simulink model "motors"  (R2021b)
settings: Solver=VariableStepAuto  StartTime=0.0  StopTime=10.0  RelTol=1e-3
values from neighbouring files (symbols this model uses):
  b = 0.2    [motor.m]
  J = 0.02    [motor.m]
  K = 0.02    [motor.m]
  L = 0.5    [motor.m]
  R = 2    [motor.m]
settings Model: Creator=Madhav R  LastModifiedBy=Madhav R

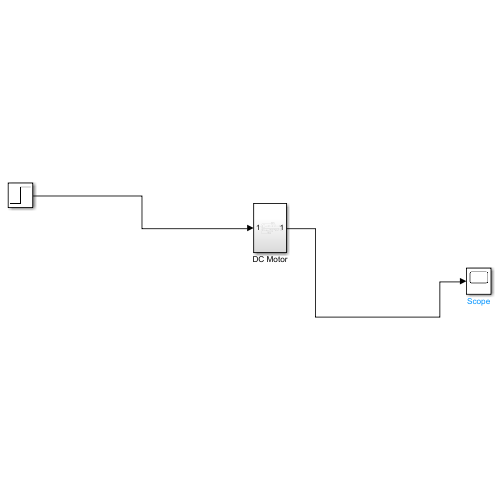
[thumbnail: Simulink's stored preview of the top-level diagram]
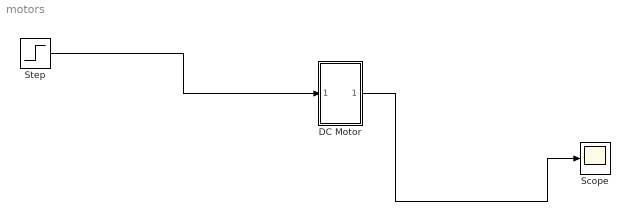
== system motors ==
  DC Motor : Subsystem
  Scope : Scope
  Step : Step  SampleTime=0
  wires:
  Step/1 -> DC Motor/1(In1)
  DC Motor/1(Out1) -> Scope/1

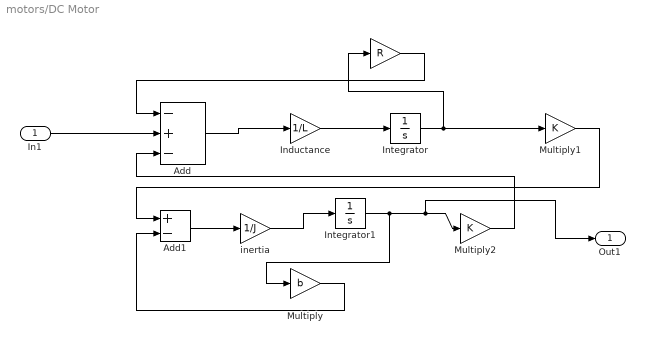
== system motors/DC Motor ==
  In1 : Inport
  " " : Gain  Gain=R
  Add : Sum  Inputs=-+-
  Add1 : Sum  Inputs=+-
  Inductance : Gain  Gain=1/L
  Integrator : Integrator
  Integrator1 : Integrator
  Multiply : Gain  Gain=b
  Multiply1 : Gain  Gain=K
  Multiply2 : Gain  Gain=K
  inertia : Gain  Gain=1/J
  Out1 : Outport
  wires:
  Multiply1/1 -> Add1/1
  Integrator1/1 -> Multiply/1, Out1/1, Multiply2/1
  Add1/1 -> inertia/1
  Inductance/1 -> Integrator/1
  Integrator/1 -> " "/1, Multiply1/1
  Add/1 -> Inductance/1
  Multiply/1 -> Add1/2
  " "/1 -> Add/1
  Multiply2/1 -> Add/3
  inertia/1 -> Integrator1/1
  In1/1 -> Add/2
